simulink model "s_c856m4k"  (R2016b)
settings: Solver=VariableStepAuto  StartTime=0.0  StopTime=10  RelTol=1e-3  EnableMultiTasking=on
undefined symbols (not defined in the file): fft_stages
libraries: xbsIndex_r4 x11811, casper_library_misc x54, casper_library_scopes x5, xps_library x2
(part 25 of 92)

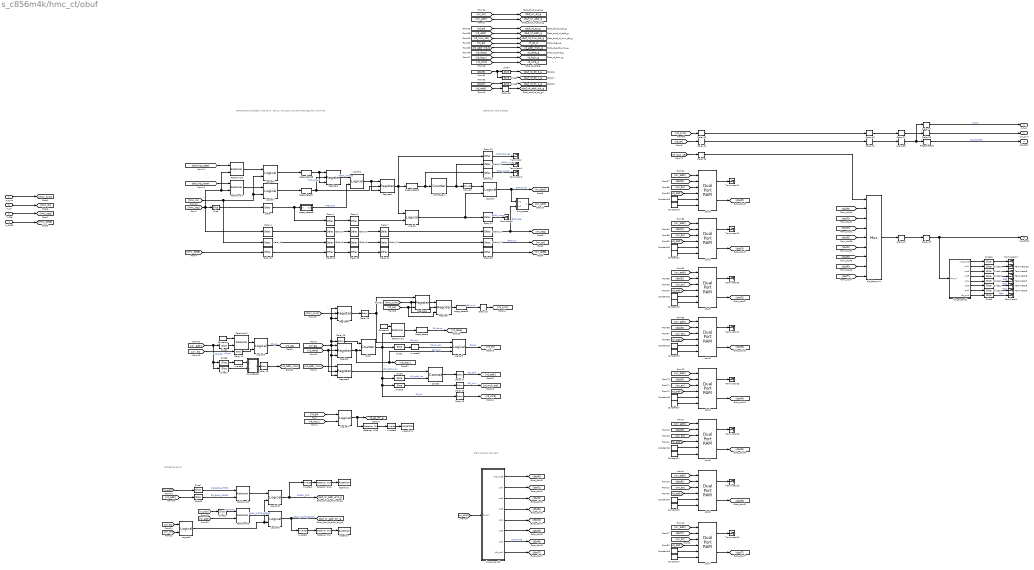
== system s_c856m4k/hmc_ct/obuf ==
  note: Addressing errors
  note: Eight parallel channels.
  note: Create the write address.
  note: Generate the corrected write bank - taking into account
      | out-of-order tags from the HMC.
  in_sync : Inport
  in_dv : Inport  Port=2
  in_tag : Inport  Port=3
  in_d256 : Inport  Port=4
  Assertion : Assertion
  Assertion1 : Assertion
  Assertion2 : Assertion
  Concat : xbsIndex_r4/Concat  num_inputs=2  dbl_ovrd=off  block_type=concat
  Constant1 : xbsIndex_r4/Constant  const=511-32  gui_display_data_type=Fixed-point  arith_type=Unsigned  n_bits=9  bin_pt=0  preci_type=Single  exp_width=8  frac_width=24  explicit_period=on  period=1  equ=P=C  opselect=C  inp2=PCIN>>17  opr=+  inp1=P  carry=CIN  dbl_ovrd=off  block_type=constant
  Constant{10,14,16,18,20,22,24,26} (8 alike) : xbsIndex_r4/Constant  const=0  gui_display_data_type=Fixed-point  arith_type=Unsigned  n_bits=256  bin_pt=0  preci_type=Single  exp_width=8  frac_width=24  explicit_period=on  period=1  equ=P=C  opselect=C  inp2=PCIN>>17  opr=+  inp1=P  carry=CIN  dbl_ovrd=off  block_type=constant
  Constant{11,15,17,19,21,23,25,27} (8 alike) : xbsIndex_r4/Constant  const=0  gui_display_data_type=Boolean  arith_type=Boolean  n_bits=256  bin_pt=0  preci_type=Single  exp_width=8  frac_width=24  explicit_period=on  period=1  equ=P=C  opselect=C  inp2=PCIN>>17  opr=+  inp1=P  carry=CIN  dbl_ovrd=off  block_type=constant
  Constant4 : xbsIndex_r4/Constant  const=0  gui_display_data_type=Fixed-point  arith_type=Unsigned  n_bits=8  bin_pt=0  preci_type=Single  exp_width=8  frac_width=24  explicit_period=on  period=1  equ=P=C  opselect=C  inp2=PCIN>>17  opr=+  inp1=P  carry=CIN  dbl_ovrd=off  block_type=constant
  Convert : xbsIndex_r4/Convert  gui_display_data_type=Boolean  arith_type=Boolean  n_bits=16  bin_pt=14  float_type=Single  exp_bits=8  fraction_bits=24  quantization=Truncate  overflow=Wrap  en=off  latency=0  pipeline=off  dbl_ovrd=off  block_type=convert
  Delay{,3..4,31} (4 alike) : xbsIndex_r4/Delay  rst=off  infoeditControl=Selection of Reset will increase slice count due to use of real FFs and instead of SRLs  en=off  latency=3  reg_retiming=off  dbl_ovrd=off  block_type=delay
      settings: infoedit=Hardware notes: A delay line is a chain, each link of which is an SRL16 or SRL32 followed by a flip-flop.
  Delay{1..2,5..12,14..23,27..29,32..35,37..38,40,45} (31 alike) : xbsIndex_r4/Delay  rst=off  infoeditControl=Selection of Reset will increase slice count due to use of real FFs and instead of SRLs  en=off  latency=1  reg_retiming=off  dbl_ovrd=off  block_type=delay
      settings: infoedit=Hardware notes: A delay line is a chain, each link of which is an SRL16 or SRL32 followed by a flip-flop.
  Delay13 : xbsIndex_r4/Delay  rst=off  infoeditControl=Selection of Reset will increase slice count due to use of real FFs and instead of SRLs  en=off  latency=2  reg_retiming=off  dbl_ovrd=off  block_type=delay
      settings: infoedit=Hardware notes: A delay line is a chain, each link of which is an SRL16 or SRL32 followed by a flip-flop.
  Delay25 : xbsIndex_r4/Delay  rst=off  infoeditControl=Selection of Reset will increase slice count due to use of real FFs and instead of SRLs  en=off  latency=pkt_buffer_latency  reg_retiming=off  dbl_ovrd=off  block_type=delay
      settings: infoedit=Hardware notes: A delay line is a chain, each link of which is an SRL16 or SRL32 followed by a flip-flop.
  Delay26 : xbsIndex_r4/Delay  rst=off  infoeditControl=Selection of Reset will increase slice count due to use of real FFs and instead of SRLs  en=off  latency=omux_latency  reg_retiming=off  dbl_ovrd=off  block_type=delay
      settings: infoedit=Hardware notes: A delay line is a chain, each link of which is an SRL16 or SRL32 followed by a flip-flop.
  Delay36 : xbsIndex_r4/Delay  rst=off  infoeditControl=Selection of Reset will increase slice count due to use of real FFs and instead of SRLs  en=off  latency=pkt_buffer_latency  reg_retiming=off  dbl_ovrd=off  block_type=delay
      settings: infoedit=Hardware notes: A delay line is a chain, each link of which is an SRL16 or SRL32 followed by a flip-flop.
  Delay42 : xbsIndex_r4/Delay  rst=off  infoeditControl=Selection of Reset will increase slice count due to use of real FFs and instead of SRLs  en=off  latency=pkt_buffer_latency  reg_retiming=off  dbl_ovrd=off  block_type=delay
      settings: infoedit=Hardware notes: A delay line is a chain, each link of which is an SRL16 or SRL32 followed by a flip-flop.
  Delay43 : xbsIndex_r4/Delay  rst=off  infoeditControl=Selection of Reset will increase slice count due to use of real FFs and instead of SRLs  en=off  latency=omux_latency  reg_retiming=off  dbl_ovrd=off  block_type=delay
      settings: infoedit=Hardware notes: A delay line is a chain, each link of which is an SRL16 or SRL32 followed by a flip-flop.
  Delay46 : xbsIndex_r4/Delay  rst=off  infoeditControl=Selection of Reset will increase slice count due to use of real FFs and instead of SRLs  en=off  latency=27  reg_retiming=off  dbl_ovrd=off  block_type=delay
      settings: infoedit=Hardware notes: A delay line is a chain, each link of which is an SRL16 or SRL32 followed by a flip-flop.
  Gateway Out : xbsIndex_r4/Gateway Out  inherit_from_input=off  hdl_port=off  rows=1  columns=1  UseAsDAC=off  DACChannel='1'  interface=None  automatic_assignment=on  address_offset=hex2dec('00')  intf_name=''  intf_description=''  timing_constraint=None  locs_specified=off  LOCs={}  io_standard={}  block_type=gatewayout
  Gateway Out1 : xbsIndex_r4/Gateway Out  inherit_from_input=off  hdl_port=off  rows=1  columns=1  UseAsDAC=off  DACChannel='1'  interface=None  automatic_assignment=on  address_offset=hex2dec('00')  intf_name=''  intf_description=''  timing_constraint=None  locs_specified=off  LOCs={}  io_standard={}  block_type=gatewayout
  Gateway Out2 : xbsIndex_r4/Gateway Out  inherit_from_input=off  hdl_port=off  rows=1  columns=1  UseAsDAC=off  DACChannel='1'  interface=None  automatic_assignment=on  address_offset=hex2dec('00')  intf_name=''  intf_description=''  timing_constraint=None  locs_specified=off  LOCs={}  io_standard={}  block_type=gatewayout
  Inverter{2..6} (5 alike) : xbsIndex_r4/Inverter  en=off  latency=0  dbl_ovrd=off  block_type=inv
  Logical{,1,3..4} (4 alike) : xbsIndex_r4/Logical  logical_function=AND  inputs=2  en=off  latency=1  precision=Full  arith_type=Unsigned  n_bits=16  bin_pt=0  align_bp=on  dbl_ovrd=off  block_type=logical
  Logical10 : xbsIndex_r4/Logical  logical_function=AND  inputs=2  en=off  latency=0  precision=Full  arith_type=Unsigned  n_bits=16  bin_pt=0  align_bp=on  dbl_ovrd=off  block_type=logical
  Logical2 : xbsIndex_r4/Logical  logical_function=XOR  inputs=2  en=off  latency=1  precision=Full  arith_type=Unsigned  n_bits=16  bin_pt=0  align_bp=on  dbl_ovrd=off  block_type=logical
  Logical5 : xbsIndex_r4/Logical  logical_function=AND  inputs=3  en=off  latency=1  precision=Full  arith_type=Unsigned  n_bits=16  bin_pt=0  align_bp=on  dbl_ovrd=off  block_type=logical
  Logical6 : xbsIndex_r4/Logical  logical_function=AND  inputs=2  en=off  latency=3  precision=Full  arith_type=Unsigned  n_bits=16  bin_pt=0  align_bp=on  dbl_ovrd=off  block_type=logical
  Logical7 : xbsIndex_r4/Logical  logical_function=AND  inputs=2  en=off  latency=3  precision=Full  arith_type=Unsigned  n_bits=16  bin_pt=0  align_bp=on  dbl_ovrd=off  block_type=logical
  Logical8 : xbsIndex_r4/Logical  logical_function=AND  inputs=2  en=off  latency=0  precision=Full  arith_type=Unsigned  n_bits=16  bin_pt=0  align_bp=on  dbl_ovrd=off  block_type=logical
  Logical9 : xbsIndex_r4/Logical  logical_function=AND  inputs=2  en=off  latency=0  precision=Full  arith_type=Unsigned  n_bits=16  bin_pt=0  align_bp=on  dbl_ovrd=off  block_type=logical
  Register{,1..4,6..7} (7 alike) : xbsIndex_r4/Register  init=0  rst=on  en=on  dbl_ovrd=off  block_type=register
  Relational1 : xbsIndex_r4/Relational  mode=a=b  op_type=Bool  en=off  latency=1  dbl_ovrd=off  block_type=relational
  Relational2 : xbsIndex_r4/Relational  mode=a=b  op_type=Bool  en=off  latency=1  dbl_ovrd=off  block_type=relational
  Relational{3,5..7} (4 alike) : xbsIndex_r4/Relational  mode=a=b  op_type=Bool  en=off  latency=0  dbl_ovrd=off  block_type=relational
  Slice : xbsIndex_r4/Slice  nbits=1  boolean_output=on  mode=Upper Bit Location + Width  bit1=0  base1=MSB of Input  bit0=0  base0=LSB of Input  dbl_ovrd=off  block_type=slice
  Slice1 : xbsIndex_r4/Slice  nbits=1  boolean_output=on  mode=Lower Bit Location + Width  bit1=0  base1=MSB of Input  bit0=5  base0=LSB of Input  dbl_ovrd=off  block_type=slice
  Slice{9..16} (8 alike) : xbsIndex_r4/Slice  nbits=9  boolean_output=off  mode=Lower Bit Location + Width  bit1=0  base1=MSB of Input  bit0=0  base0=LSB of Input  dbl_ovrd=off  block_type=slice
  Slice17 : xbsIndex_r4/Slice  nbits=1  boolean_output=off  mode=Upper Bit Location + Width  bit1=-1  base1=MSB of Input  bit0=0  base0=LSB of Input  dbl_ovrd=off  block_type=slice
  Slice18 : xbsIndex_r4/Slice  nbits=2  boolean_output=off  mode=Upper Bit Location + Width  bit1=0  base1=MSB of Input  bit0=8 - 3  base0=LSB of Input  dbl_ovrd=off  block_type=slice
  Slice19 : xbsIndex_r4/Slice  nbits=3  boolean_output=off  mode=Lower Bit Location + Width  bit1=0  base1=MSB of Input  bit0=5+1  base0=LSB of Input  dbl_ovrd=off  block_type=slice
  Slice2 : xbsIndex_r4/Slice  nbits=8  boolean_output=off  mode=Lower Bit Location + Width  bit1=0  base1=MSB of Input  bit0=0  base0=LSB of Input  dbl_ovrd=off  block_type=slice
  Slice21 : xbsIndex_r4/Slice  nbits=1  boolean_output=off  mode=Two Bit Locations  bit1=0  base1=MSB of Input  bit0=3  base0=LSB of Input  dbl_ovrd=off  block_type=slice
  Slice3 : xbsIndex_r4/Slice  nbits=5  boolean_output=off  mode=Lower Bit Location + Width  bit1=0  base1=MSB of Input  bit0=0  base0=LSB of Input  dbl_ovrd=off  block_type=slice
  Slice4 : xbsIndex_r4/Slice  nbits=12  boolean_output=off  mode=Lower Bit Location + Width  bit1=0  base1=MSB of Input  bit0=0  base0=LSB of Input  dbl_ovrd=off  block_type=slice
  Slice5 : xbsIndex_r4/Slice  nbits=12  boolean_output=off  mode=Lower Bit Location + Width  bit1=0  base1=MSB of Input  bit0=32*7  base0=LSB of Input  dbl_ovrd=off  block_type=slice
  Slice6 : xbsIndex_r4/Slice  nbits=12  boolean_output=off  mode=Lower Bit Location + Width  bit1=0  base1=MSB of Input  bit0=32  base0=LSB of Input  dbl_ovrd=off  block_type=slice
  Slice7 : xbsIndex_r4/Slice  nbits=2  boolean_output=off  mode=Upper Bit Location + Width  bit1=0  base1=MSB of Input  bit0=0  base0=LSB of Input  dbl_ovrd=off  block_type=slice
  Slice8 : xbsIndex_r4/Slice  nbits=1  boolean_output=off  mode=Upper Bit Location + Width  bit1=0  base1=MSB of Input  bit0=0  base0=LSB of Input  dbl_ovrd=off  block_type=slice
  Terminator{,1..19} (20 alike) : Terminator
  WRITE_bank : xbsIndex_r4/Counter  cnt_type=Free Running  cnt_to=Inf  operation=Up  start_count=0  cnt_by_val=1  arith_type=Unsigned  n_bits=1  bin_pt=0  load_pin=off  rst=off  en=on  explicit_period=on  period=1  use_behavioral_HDL=off  implementation=Fabric  dbl_ovrd=off  block_type=counter
  bus_create : Subsystem  AncestorBlock=casper_library_flow_control/bus_create  mask(bus_create){inputNum=2}
      mask prompts: inputNum "Number of inputs:"
      mask init:
      | bus_create_init(gcb,...
      |     'inputNum', inputNum);
  bus_create1 : Subsystem  AncestorBlock=casper_library_flow_control/bus_create  mask(bus_create){inputNum=2}
      mask prompts: inputNum "Number of inputs:"
      mask init:
      | bus_create_init(gcb,...
      |     'inputNum', inputNum);
  bus_expand2 : Subsystem  AncestorBlock=casper_library_flow_control/bus_expand  mask(bus_expand){mode=divisions of equal size, outputNum=8, outputWidth=32, outputBinaryPt=0, outputArithmeticType=0, show_format=on, outputToWorkspace=off, variablePrefix=out, outputToModelAsWell=on}
      mask prompts: outputNum "Number of outputs:"; outputWidth "Output width:"; outputBinaryPt "Output binary point position:"; outputArithmeticType "Output arithmetic type (ufix=0, fix=1, bool=2):"; show_format "Print format string?"; outputToWorkspace "Output to workspace?"; variablePrefix "Variable name prefix:"; outputToModelAsWell "Output to model as well?"
      mask help:
      | Expands a 'bus' made using a bus_create or Xilinx
      | concat block.
      | The input will be divided into the specified number
      | of outputs with the specified arithmetic types.
      | Divisions are made from most significant bit.
      mask init: same as s_c856m4k/bus_expand
      settings: AttributesFormatString=8 outputs: uf32.0,uf32.0,uf32.0,uf32.0,uf32.0,uf32.0,uf32.0,uf32.0,
      mask TypeOptions mode: divisions of equal size | divisions of arbitrary size
      mask Callback mode: bus_expand_callback();
      mask Callback outputWidth: bus_expand_callback();
      mask Callback outputToWorkspace: bus_expand_callback();
  bus_expand3 : Subsystem  AncestorBlock=casper_library_flow_control/bus_expand  mask(bus_expand){mode=divisions of equal size, outputNum=8, outputWidth=32, outputBinaryPt=0, outputArithmeticType=0, show_format=off, outputToWorkspace=off, variablePrefix=out, outputToModelAsWell=on}
      mask prompts: outputNum "Number of outputs:"; outputWidth "Output width:"; outputBinaryPt "Output binary point position:"; outputArithmeticType "Output arithmetic type (ufix=0, fix=1, bool=2):"; show_format "Print format string?"; outputToWorkspace "Output to workspace?"; variablePrefix "Variable name prefix:"; outputToModelAsWell "Output to model as well?"
      mask help:
      | Expands a 'bus' made using a bus_create or Xilinx
      | concat block.
      | The input will be divided into the specified number
      | of outputs with the specified arithmetic types.
      | Divisions are made from most significant bit.
      mask init: same as s_c856m4k/bus_expand
      settings: AttributesFormatString=8 outputs
      mask TypeOptions mode: divisions of equal size | divisions of arbitrary size
      mask Callback mode: bus_expand_callback();
      mask Callback outputWidth: bus_expand_callback();
      mask Callback outputToWorkspace: bus_expand_callback();
  edge_detect{,1,3,6..8} (6 alike) : casper_library_misc/edge_detect  edge=Rising  polarity=Active High  x_in=[0 0.08 0.08 0.16 0.16 0.24 0.24 0.32 0.32 0.4]  y_in="[-1 -1  1  1  1  1  1  1  1  1]"  x_out=[0.6 0.68 0.68 0.76 0.76 0.84 0.84 0.92 0.92 1]  y_out="[-1 -1  1  1 -1 -1 -1 -1 -1 -1]"
  edge_detect5 : Subsystem  AncestorBlock=casper_library_misc/edge_detect  mask(edge_detect){edge=Falling, polarity=Active High, x_in=[0 0.08 0.08 0.16 0.16 0.24 0.24 0.32 0.32 0.4], y_in=[-1 -1  1  1  1  1  1  1  1  1], x_out=[0.6 0.68 0.68 0.76 0.76 0.84 0.84 0.92 0.92 1], y_out=[-1 -1  1  1 -1 -1 -1 -1 -1 -1]}
      mask prompts: edge "Edge Type"; polarity "Output Polarity"; x_in "Input X Positions"; y_in "Input Y Positions"; x_out "Output X Positions"; y_out "Output Y Positions"
      mask help: Output is active for one-cycle after each edge of the specified type (i.e. rising, falling or both).
      mask init: same as s_c856m4k/edge_detect1
      settings: AttributesFormatString=|
      | falling edges
      | active high
      mask Help: Output is active for one-cycle after each edge of the specified type (i.e. rising, falling, or both).  Latency is zero.
      mask TypeOptions edge: Rising | Falling | Both
      mask TypeOptions polarity: Active High | Active Low
      mask Display:
      | plot(x_in_num,0.5+y_in_num*0.2);
      | plot(x_out_num,0.5+y_out_num*0.2);
  obuf{0..7} (8 alike) : xbsIndex_r4/Dual Port RAM  depth=2^(output_len_bits + 2)  initVector=zeros(1, 2^(output_len_bits + 2))  distributed_mem=Block RAM  init_a=0  init_b=0  rst_a=off  rst_b=off  en_a=off  en_b=off  latency=pkt_buffer_latency  write_mode_A=Read After Write  write_mode_B=Read After Write  optimize=Area  dbl_ovrd=off  block_type=dpram
  pkt_data_mux : xbsIndex_r4/Mux  inputs=8  en=off  latency=omux_latency  precision=Full  arith_type=Unsigned  n_bits=16  bin_pt=14  quantization=Truncate  overflow=Wrap  dbl_ovrd=off  block_type=mux
  rd_ctr : xbsIndex_r4/Counter  cnt_type=Free Running  cnt_to=Inf  operation=Up  start_count=0  cnt_by_val=1  arith_type=Unsigned  n_bits=9  bin_pt=0  load_pin=off  rst=on  en=on  explicit_period=on  period=1  use_behavioral_HDL=off  implementation=Fabric  dbl_ovrd=off  block_type=counter
  out_sync : Outport
  out_dv : Outport  Port=2
  out_d256 : Outport  Port=3
  pkt_start : Outport  Port=4
  tag scope: obuf_ct_addr_err2_g=global, obuf_ct_addr_err_g=global, obuf_rd_addr_g=global, obuf_rd_addr_out_g=global, obuf_rd_d0_0_g=global, obuf_rd_d0_7_g=global, obuf_rd_d7_1_g=global, obuf_rd_en_g=global, obuf_rd_mux_sel_g=global, obuf_wr_addr_g=global, obuf_wr_en_g=global, rd_addr_msw_g=global, rd_busy_g=global, rd_ctr9_g=global, rd_done_g=global, rd_go_err_g=global, rd_go_g=global
  wires:
  Delay28/1 -> out_sync/1
  Delay27/1 -> Delay28/1
  Delay26/1 -> Delay27/1
  Delay25/1 -> Delay26/1
  [rd_sync] -> Delay25/1
  Delay29/1 -> [rd_sync]
  [rd_go] -> Register6/3, Register7/3
  [hmc_sync] -> Register6/2, Register7/2
  edge_detect3/1 -> Delay29/1  "RD_sync"
  Register7/1 -> edge_detect3/1
  Register6/1 -> Register7/1
  Delay19/1 -> Logical5/1, Register6/1  "RD_arm"
  Register4/1 -> Delay19/1
  [hmc_sync] -> Register4/2
  Gateway Out2/1 -> Inverter6/1
  Inverter6/1 -> Assertion2/1
  [rd_en] -> [obuf_rd_en_g]
  Delay15/1 -> [rd_ctr9]
  [rd_ctr9] -> [rd_ctr9_g]
  [rd_busy] -> [rd_busy_g]
  [rd_done] -> [rd_done_g]
  [rd_addr_msw] -> [rd_addr_msw_g]
  [rd_go] -> [rd_go_g]
  Slice19/1 -> Delay18/1
  Delay18/1 -> [rd_mux_sel]  "RD_mux"
  Delay17/1 -> [rd_addr]  "RD_addr"
  Logical5/1 -> [rd_en]  "RD_en"
  Concat/1 -> Delay17/1
  [rd_done] -> Register/2, Register3/2
  edge_detect/1 -> [rd_done]  "RD_done"
  Relational1/1 -> edge_detect/1
  Constant1/1 -> Relational1/1
  Register3/1 -> Concat/1  "RD_addr_msw"
  [rd_addr_msw] -> Register3/1
  Slice3/1 -> Concat/2  "RD_addr_lsw"
  Inverter5/1 -> Logical5/2  "RD_en_raw"
  Slice1/1 -> Inverter5/1
  rd_ctr/1 -> Relational1/2, Slice3/1, Slice19/1, Delay15/1, Slice1/1  "RD_ctr"
  Delay16/1 -> rd_ctr/1
  Register/1 -> [rd_busy], Logical5/3, rd_ctr/2  "RD_busy"
  [rd_go] -> Register/1, Register/3, Register3/3, Delay16/1, Register4/1, Register4/3
  Logical4/1 -> [rd_go_err_g], Gateway Out2/1
  [rd_busy] -> Logical4/2
  [rd_go] -> Logical4/1
  Delay13/1 -> [rd_addr_msw]
  Logical3/1 -> [rd_go]  "RD_go"
  Delay14/1 -> Logical3/2
  Slice17/1 -> bus_create1/2(in2)
  Inverter3/1 -> bus_create1/1(in1)
  bus_create1/1(bus_out) -> Delay13/1
  Slice8/1 -> Inverter3/1
  [wr_addr] -> Slice17/1, Slice8/1, Slice2/1  "WR_addr"
  Slice2/1 -> Relational2/2
  [wr_en] -> Delay14/1  "WR_en"
  Relational2/1 -> Logical3/1
  Constant4/1 -> Relational2/1
  Delay46/1 -> [obuf_rd_addr_out_g]
  [rd_addr] -> Delay46/1
  Slice6/1 -> [obuf_rd_d7_1_g]
  [obuf7] -> Slice6/1
  Slice5/1 -> [obuf_rd_d0_7_g]
  Slice4/1 -> [obuf_rd_d0_0_g]
  [obuf0] -> Slice4/1, Slice5/1
  [rd_mux_sel] -> [obuf_rd_mux_sel_g]
  [rd_addr] -> [obuf_rd_addr_g]
  [wr_addr] -> [obuf_wr_addr_g]
  [wr_en] -> [obuf_wr_en_g]
  Inverter4/1 -> Gateway Out1/1
  Gateway Out1/1 -> Assertion1/1
  Logical10/1 -> [obuf_ct_addr_err2_g], Inverter4/1  "CHECK_DIFF"
  Relational5/1 -> Logical8/1  "READ_WRITE_ERROR"
  Relational3/1 -> Logical10/1
  Slice18/1 -> Relational3/2  "RD_BANK_CHECK"
  Slice7/1 -> Relational3/1  "WR_BANK_CHECK"
  [rd_addr] -> Slice18/1
  [wr_addr] -> Slice7/1
  Logical9/1 -> Logical8/2, Logical10/2
  Slice21/1 -> Relational5/1  "WADDR7"
  Inverter2/1 -> Gateway Out/1
  Gateway Out/1 -> Assertion/1
  [wr_en] -> Logical9/2
  [rd_en] -> Logical9/1
  Logical8/1 -> Inverter2/1, [obuf_ct_addr_err_g]  "READ_WRITE_ERROR"
  [rd_addr] -> Relational5/2
  [wr_addr] -> Slice21/1
  bus_expand3/8(lsb_out1) -> [dbuf7]
  bus_expand3/7(out2) -> [dbuf6]  "DATA_TAG"
  bus_expand3/6(out3) -> [dbuf5]
  bus_expand3/5(out4) -> [dbuf4]
  bus_expand3/4(out5) -> [dbuf3]
  bus_expand3/3(out6) -> [dbuf2]
  bus_expand3/2(out7) -> [dbuf1]
  bus_expand3/1(msb_out8) -> [dbuf0]
  [wr_d256] -> bus_expand3/1(bus_in)
  Delay40/1 -> Delay45/1
  Delay38/1 -> edge_detect1/1, Delay37/1
  Delay37/1 -> out_dv/1  "out_dv"
  Delay45/1 -> bus_expand2/1(bus_in), out_d256/1
  edge_detect1/1 -> pkt_start/1  "out_pkt_start"
  Delay43/1 -> Delay38/1
  Delay42/1 -> Delay43/1
  [rd_en] -> Delay42/1
  Delay36/1 -> pkt_data_mux/1
  [obuf1] -> pkt_data_mux/3
  [obuf0] -> pkt_data_mux/2
  [obuf2] -> pkt_data_mux/4
  [obuf3] -> pkt_data_mux/5
  [obuf7] -> pkt_data_mux/9
  [obuf5] -> pkt_data_mux/7
  [obuf6] -> pkt_data_mux/8
  [obuf4] -> pkt_data_mux/6
  [rd_mux_sel] -> Delay36/1
  obuf4/1 -> Terminator15/1
  obuf4/2 -> [obuf4]
  Constant27/1 -> obuf4/6
  Constant26/1 -> obuf4/5
  [rd_addr] -> obuf4/4
  [wr_en] -> obuf4/3
  [wr_addr] -> obuf4/1
  [dbuf4] -> obuf4/2
  obuf3/1 -> Terminator14/1
  obuf3/2 -> [obuf3]
  Constant25/1 -> obuf3/6
  Constant24/1 -> obuf3/5
  [rd_addr] -> obuf3/4
  [wr_en] -> obuf3/3
  [wr_addr] -> obuf3/1
  [dbuf3] -> obuf3/2
  obuf2/1 -> Terminator13/1
  obuf2/2 -> [obuf2]
  Constant23/1 -> obuf2/6
  Constant22/1 -> obuf2/5
  [rd_addr] -> obuf2/4
  [wr_en] -> obuf2/3
  [wr_addr] -> obuf2/1
  [dbuf2] -> obuf2/2
  obuf1/1 -> Terminator12/1
  obuf1/2 -> [obuf1]
  Constant21/1 -> obuf1/6
  Constant20/1 -> obuf1/5
  [rd_addr] -> obuf1/4
  [wr_en] -> obuf1/3
  [wr_addr] -> obuf1/1
  [dbuf1] -> obuf1/2
  obuf0/1 -> Terminator11/1
  obuf0/2 -> [obuf0]
  Constant19/1 -> obuf0/6
  Constant18/1 -> obuf0/5
  [rd_addr] -> obuf0/4
  [wr_en] -> obuf0/3
  [wr_addr] -> obuf0/1
  [dbuf0] -> obuf0/2
  obuf7/1 -> Terminator10/1
  obuf7/2 -> [obuf7]
  Constant17/1 -> obuf7/6
  Constant16/1 -> obuf7/5
  [rd_addr] -> obuf7/4
  [wr_en] -> obuf7/3
  [wr_addr] -> obuf7/1
  [dbuf7] -> obuf7/2
  obuf6/1 -> Terminator19/1
  obuf6/2 -> [obuf6]
  Constant15/1 -> obuf6/6
  Constant14/1 -> obuf6/5
  [rd_addr] -> obuf6/4
  [wr_en] -> obuf6/3
  [wr_addr] -> obuf6/1
  [dbuf6] -> obuf6/2
  pkt_data_mux/1 -> Delay40/1
  obuf5/1 -> Terminator18/1
  obuf5/2 -> [obuf5]
  bus_expand2/4(out5) -> Slice13/1
  Slice13/1 -> Terminator8/1
  Slice14/1 -> Terminator9/1
  Slice15/1 -> Terminator16/1
  Slice16/1 -> Terminator17/1
  bus_expand2/3(out6) -> Slice14/1
  bus_expand2/2(out7) -> Slice15/1
  bus_expand2/1(msb_out8) -> Slice16/1
  Slice9/1 -> Terminator4/1  "tag0"
  Slice10/1 -> Terminator5/1  "tag1"
  Slice11/1 -> Terminator6/1  "tag2"
  Slice12/1 -> Terminator7/1  "tag3"
  bus_expand2/5(out4) -> Slice12/1
  bus_expand2/6(out3) -> Slice11/1
  bus_expand2/7(out2) -> Slice10/1
  bus_expand2/8(lsb_out1) -> Slice9/1
  Constant11/1 -> obuf5/6
  Constant10/1 -> obuf5/5
  [rd_addr] -> obuf5/4
  [wr_en] -> obuf5/3
  [wr_addr] -> obuf5/1
  [dbuf5] -> obuf5/2
  Delay35/1 -> [wr_d256]
  Delay34/1 -> Delay35/1
  Delay33/1 -> Delay34/1
  Delay32/1 -> Delay33/1
  Delay31/1 -> Delay32/1
  [hmc_d256] -> Delay31/1
  in_d256/1 -> [hmc_d256]
  edge_detect8/1 -> WRITE_bank/1, Delay21/1
  Register1/1 -> edge_detect8/1, Logical/1, Delay23/1
  Delay23/1 -> Terminator/1  "BANK_change"
  Delay22/1 -> Terminator3/1  "BANK_wrong"
  Delay21/1 -> Terminator2/1  "BANK_switch"
  Delay20/1 -> Terminator1/1  "BANK_wr_raw"
  Delay3/1 -> Delay8/1
  Delay8/1 -> Delay9/1
  Delay9/1 -> Delay10/1
  Delay10/1 -> Delay11/1
  Delay11/1 -> [wr_en]  "BANK_dv"
  Delay12/1 -> bus_create/2(in2), [wr_tag]  "BANK_tag"
  bus_create/1(bus_out) -> [wr_addr]
  Logical2/1 -> bus_create/1(in1), [wr_bank]  "BANK_final"
  Delay2/1 -> Logical/2
  Logical/1 -> Logical2/2, Delay22/1
  Delay7/1 -> Delay12/1
  Delay6/1 -> Delay7/1
  Delay5/1 -> Delay6/1
  Delay4/1 -> Delay5/1
  Convert/1 -> Logical2/1
  Delay1/1 -> Delay2/1
  WRITE_bank/1 -> Convert/1, Delay20/1
  Logical1/1 -> Register1/1, Register1/3
  Register2/1 -> Logical1/1  "BANK_change"
  edge_detect7/1 -> Register2/2, Register1/2
  [hmc_dv] -> Delay3/1, Logical7/2, Logical6/2
  [obuf_trig_lower] -> Relational7/1
  edge_detect6/1 -> Register2/1, Register2/3  "TAG_upper"
  Relational6/1 -> Logical6/1
  [obuf_trig_upper] -> Relational6/1
  Delay/1 -> edge_detect5/1(in), Delay1/1
  edge_detect5/1(out) -> Logical1/2  "TAG_drop"
  Slice/1 -> Delay/1
  [hmc_tag] -> Slice/1, Delay4/1, Relational7/2, Relational6/2
  in_sync/1 -> [hmc_sync]
  in_tag/1 -> [hmc_tag]
  in_dv/1 -> [hmc_dv]
  Relational7/1 -> Logical7/1
  Logical6/1 -> edge_detect6/1
  Logical7/1 -> edge_detect7/1

== system s_c856m4k/hmc_ct/read_map_gen_interleave ==
  note: collection of like channels
  note: Straight collection, no x-interleave
  note: x-interleave, SLICED
  note: x-interleave, CALCED
  note: compare calculated to sliced
  addr : Inport
  num_x : Inport  Port=2
  one_over_num_x : Inport  Port=3
  chans_per_x_div8 : Inport  Port=4
  AddSub2 : xbsIndex_r4/AddSub  mode=Subtraction  use_carryin=off  use_carryout=off  en=off  latency=0  precision=Full  arith_type=Unsigned  n_bits=7  bin_pt=0  quantization=Truncate  overflow=Wrap  use_behavioral_HDL=off  hw_selection=Fabric  pipelined=off  dbl_ovrd=off  block_type=addsub
  AddSub3 : xbsIndex_r4/AddSub  mode=Subtraction  use_carryin=off  use_carryout=off  en=off  latency=3  precision=User Defined  arith_type=Unsigned  n_bits=in_vec_bits - 2  bin_pt=0  quantization=Truncate  overflow=Wrap  use_behavioral_HDL=off  hw_selection=Fabric  pipelined=off  dbl_ovrd=off  block_type=addsub
  AddSub4 : xbsIndex_r4/AddSub  mode=Addition  use_carryin=off  use_carryout=off  en=off  latency=3  precision=User Defined  arith_type=Unsigned  n_bits=in_vec_bits  bin_pt=0  quantization=Truncate  overflow=Wrap  use_behavioral_HDL=off  hw_selection=Fabric  pipelined=off  dbl_ovrd=off  block_type=addsub
  Assert1 : xbsIndex_r4/Assert  assert_type=on  type_source=Explicitly  gui_display_data_type=Fixed-point  arith_type=Unsigned  n_bits=in_vec_bits  bin_pt=0  preci_type=Single  exp_width=8  frac_width=24  assert_rate=on  rate_source=Explicitly  period=1  output_port=on  block_type=assert
  Assert{2,6..9} (5 alike) : xbsIndex_r4/Assert  assert_type=on  type_source=Explicitly  gui_display_data_type=Fixed-point  arith_type=Unsigned  n_bits=in_vec_bits + out_vec_bits + 1  bin_pt=0  preci_type=Single  exp_width=8  frac_width=24  assert_rate=on  rate_source=Explicitly  period=1  output_port=on  block_type=assert
  Assert3 : xbsIndex_r4/Assert  assert_type=on  type_source=Explicitly  gui_display_data_type=Fixed-point  arith_type=Unsigned  n_bits=8  bin_pt=0  preci_type=Single  exp_width=8  frac_width=24  assert_rate=on  rate_source=Explicitly  period=1  output_port=on  block_type=assert
  Assert4 : xbsIndex_r4/Assert  assert_type=on  type_source=Explicitly  gui_display_data_type=Fixed-point  arith_type=Unsigned  n_bits=9  bin_pt=8  preci_type=Single  exp_width=8  frac_width=24  assert_rate=on  rate_source=Explicitly  period=1  output_port=on  block_type=assert
  Assert5 : xbsIndex_r4/Assert  assert_type=on  type_source=Explicitly  gui_display_data_type=Fixed-point  arith_type=Unsigned  n_bits=12  bin_pt=0  preci_type=Single  exp_width=8  frac_width=24  assert_rate=on  rate_source=Explicitly  period=1  output_port=on  block_type=assert
  Assertion : Assertion
  Concat1 : xbsIndex_r4/Concat  num_inputs=3  dbl_ovrd=off  block_type=concat
  Concat10 : xbsIndex_r4/Concat  num_inputs=3  dbl_ovrd=off  block_type=concat
  Concat4 : xbsIndex_r4/Concat  num_inputs=3  dbl_ovrd=off  block_type=concat
  Concat8 : xbsIndex_r4/Concat  num_inputs=2  dbl_ovrd=off  block_type=concat
  Mult3 : xbsIndex_r4/Mult  precision=User Defined  arith_type=Unsigned  n_bits=in_vec_bits - 1 + 8  bin_pt=0  quantization=Truncate  overflow=Wrap  en=off  latency=3  use_behavioral_HDL=off  opt=Speed  use_embedded=on  optimum_pipeline=off  pipeline=on  dbl_ovrd=off  use_rpm=on  placement_style=Triangular  block_type=mult
  Mult4 : xbsIndex_r4/Mult  precision=User Defined  arith_type=Unsigned  n_bits=in_vec_bits + 8  bin_pt=0  quantization=Truncate  overflow=Wrap  en=off  latency=3  use_behavioral_HDL=off  opt=Speed  use_embedded=on  optimum_pipeline=off  pipeline=on  dbl_ovrd=off  use_rpm=on  placement_style=Triangular  block_type=mult
  Mult5 : xbsIndex_r4/Mult  precision=User Defined  arith_type=Unsigned  n_bits=in_vec_bits - 1 + 8  bin_pt=0  quantization=Truncate  overflow=Wrap  en=off  latency=3  use_behavioral_HDL=off  opt=Speed  use_embedded=on  optimum_pipeline=off  pipeline=on  dbl_ovrd=off  use_rpm=on  placement_style=Triangular  block_type=mult
  Relational : xbsIndex_r4/Relational  mode=a=b  op_type=Bool  en=off  latency=0  dbl_ovrd=off  block_type=relational
  Terminator{,1..7} (8 alike) : Terminator
  bank1 : xbsIndex_r4/Slice  nbits=x_bits  boolean_output=off  mode=Upper Bit Location + Width  bit1=0  base1=MSB of Input  bit0=0  base0=LSB of Input  dbl_ovrd=off  block_type=slice
  bank10 : xbsIndex_r4/Slice  nbits=in_vec_bits  boolean_output=off  mode=Lower Bit Location + Width  bit1=2  base1=MSB of Input  bit0=out_vec_bits  base0=LSB of Input  dbl_ovrd=off  block_type=slice
  bank11 : xbsIndex_r4/Slice  nbits=out_vec_bits  boolean_output=off  mode=Lower Bit Location + Width  bit1=2  base1=MSB of Input  bit0=0  base0=LSB of Input  dbl_ovrd=off  block_type=slice
  bank12 : xbsIndex_r4/Slice  nbits=1  boolean_output=off  mode=Upper Bit Location + Width  bit1=0  base1=MSB of Input  bit0=output_len_bits - 1  base0=LSB of Input  dbl_ovrd=off  block_type=slice
  bank2 : xbsIndex_r4/Slice  nbits=x_bits  boolean_output=off  mode=Upper Bit Location + Width  bit1=0  base1=MSB of Input  bit0=0  base0=LSB of Input  dbl_ovrd=off  block_type=slice
  bank23 : xbsIndex_r4/Slice  nbits=x_bits  boolean_output=off  mode=Lower Bit Location + Width  bit1=2  base1=MSB of Input  bit0=0  base0=LSB of Input  dbl_ovrd=off  block_type=slice
  bank25 : xbsIndex_r4/Slice  nbits=x_bits  boolean_output=off  mode=Two Bit Locations  bit1=0  base1=MSB of Input  bit0=x_bits  base0=LSB of Input  dbl_ovrd=off  block_type=slice
  bank3 : xbsIndex_r4/Slice  nbits=out_vec_bits  boolean_output=off  mode=Lower Bit Location + Width  bit1=2  base1=MSB of Input  bit0=in_vec_bits  base0=LSB of Input  dbl_ovrd=off  block_type=slice
  bank4 : xbsIndex_r4/Slice  nbits=out_vec_bits  boolean_output=off  mode=Lower Bit Location + Width  bit1=2  base1=MSB of Input  bit0=in_vec_bits  base0=LSB of Input  dbl_ovrd=off  block_type=slice
  bank5 : xbsIndex_r4/Slice  nbits=in_vec_bits  boolean_output=off  mode=Lower Bit Location + Width  bit1=2  base1=MSB of Input  bit0=0  base0=LSB of Input  dbl_ovrd=off  block_type=slice
  bank6 : xbsIndex_r4/Slice  nbits=in_vec_bits  boolean_output=off  mode=Lower Bit Location + Width  bit1=2  base1=MSB of Input  bit0=0  base0=LSB of Input  dbl_ovrd=off  block_type=slice
  bank7 : xbsIndex_r4/Slice  nbits=x_bits  boolean_output=off  mode=Upper Bit Location + Width  bit1=0  base1=MSB of Input  bit0=0  base0=LSB of Input  dbl_ovrd=off  block_type=slice
  bank8 : xbsIndex_r4/Slice  nbits=out_vec_bits  boolean_output=off  mode=Lower Bit Location + Width  bit1=2  base1=MSB of Input  bit0=in_vec_bits  base0=LSB of Input  dbl_ovrd=off  block_type=slice
  bank9 : xbsIndex_r4/Slice  nbits=in_vec_bits  boolean_output=off  mode=Lower Bit Location + Width  bit1=2  base1=MSB of Input  bit0=0  base0=LSB of Input  dbl_ovrd=off  block_type=slice
  chans_per_x1 : xbsIndex_r4/Constant  const=0  gui_display_data_type=Fixed-point  arith_type=Signed (2's comp)  n_bits=15  bin_pt=0  preci_type=Single  exp_width=8  frac_width=24  explicit_period=on  period=1  equ=P=C  opselect=C  inp2=PCIN>>17  opr=+  inp1=P  carry=CIN  dbl_ovrd=off  block_type=constant
  in_vec_len : xbsIndex_r4/Constant  const=2^in_vec_bits  gui_display_data_type=Fixed-point  arith_type=Unsigned  n_bits=in_vec_bits + 1  bin_pt=0  preci_type=Single  exp_width=8  frac_width=24  explicit_period=on  period=1  equ=P=C  opselect=C  inp2=PCIN>>17  opr=+  inp1=P  carry=CIN  dbl_ovrd=off  block_type=constant
  out_vec_len : xbsIndex_r4/Constant  const=2^out_vec_bits  gui_display_data_type=Fixed-point  arith_type=Unsigned  n_bits=out_vec_bits + 1  bin_pt=0  preci_type=Single  exp_width=8  frac_width=24  explicit_period=on  period=1  equ=P=C  opselect=C  inp2=PCIN>>17  opr=+  inp1=P  carry=CIN  dbl_ovrd=off  block_type=constant
  we_delay1 : Subsystem  AncestorBlock=casper_library_delays/pipeline  mask(pipeline){latency=3}
      mask help:
      | An explicitly laid-out delay line to avoid mapping to SRL16s
      | for use in pipelining to help achieve timing closure.
      mask init:
      | pipeline_init(gcb,'latency',latency);
      settings: AttributesFormatString=Latency = %<latency>
      mask Display:
      | port_label('input', 1, 'd');
      | port_label('output', 1, 'q');
      | disp(['Z^-', num2str(latency)]);
  we_delay10 : Subsystem  AncestorBlock=casper_library_delays/pipeline  mask(pipeline){latency=3}
      mask help:
      | An explicitly laid-out delay line to avoid mapping to SRL16s
      | for use in pipelining to help achieve timing closure.
      mask init:
      | pipeline_init(gcb,'latency',latency);
      settings: AttributesFormatString=Latency = %<latency>
      mask Display:
      | port_label('input', 1, 'd');
      | port_label('output', 1, 'q');
      | disp(['Z^-', num2str(latency)]);
  we_delay11 : Subsystem  AncestorBlock=casper_library_delays/pipeline  mask(pipeline){latency=3}
      mask help:
      | An explicitly laid-out delay line to avoid mapping to SRL16s
      | for use in pipelining to help achieve timing closure.
      mask init:
      | pipeline_init(gcb,'latency',latency);
      settings: AttributesFormatString=Latency = %<latency>
      mask Display:
      | port_label('input', 1, 'd');
      | port_label('output', 1, 'q');
      | disp(['Z^-', num2str(latency)]);
  we_delay12 : Subsystem  AncestorBlock=casper_library_delays/pipeline  mask(pipeline){latency=3}
      mask help:
      | An explicitly laid-out delay line to avoid mapping to SRL16s
      | for use in pipelining to help achieve timing closure.
      mask init:
      | pipeline_init(gcb,'latency',latency);
      settings: AttributesFormatString=Latency = %<latency>
      mask Display:
      | port_label('input', 1, 'd');
      | port_label('output', 1, 'q');
      | disp(['Z^-', num2str(latency)]);
  we_delay13 : Subsystem  AncestorBlock=casper_library_delays/pipeline  mask(pipeline){latency=3}
      mask help:
      | An explicitly laid-out delay line to avoid mapping to SRL16s
      | for use in pipelining to help achieve timing closure.
      mask init:
      | pipeline_init(gcb,'latency',latency);
      settings: AttributesFormatString=Latency = %<latency>
      mask Display:
      | port_label('input', 1, 'd');
      | port_label('output', 1, 'q');
      | disp(['Z^-', num2str(latency)]);
  we_delay14 : Subsystem  AncestorBlock=casper_library_delays/pipeline  mask(pipeline){latency=3}
      mask help:
      | An explicitly laid-out delay line to avoid mapping to SRL16s
      | for use in pipelining to help achieve timing closure.
      mask init:
      | pipeline_init(gcb,'latency',latency);
      settings: AttributesFormatString=Latency = %<latency>
      mask Display:
      | port_label('input', 1, 'd');
      | port_label('output', 1, 'q');
      | disp(['Z^-', num2str(latency)]);
  we_delay15 : Subsystem  AncestorBlock=casper_library_delays/pipeline  mask(pipeline){latency=3}
      mask help:
      | An explicitly laid-out delay line to avoid mapping to SRL16s
      | for use in pipelining to help achieve timing closure.
      mask init:
      | pipeline_init(gcb,'latency',latency);
      settings: AttributesFormatString=Latency = %<latency>
      mask Display:
      | port_label('input', 1, 'd');
      | port_label('output', 1, 'q');
      | disp(['Z^-', num2str(latency)]);
  we_delay16 : Subsystem  AncestorBlock=casper_library_delays/pipeline  mask(pipeline){latency=3}
      mask help:
      | An explicitly laid-out delay line to avoid mapping to SRL16s
      | for use in pipelining to help achieve timing closure.
      mask init:
      | pipeline_init(gcb,'latency',latency);
      settings: AttributesFormatString=Latency = %<latency>
      mask Display:
      | port_label('input', 1, 'd');
      | port_label('output', 1, 'q');
      | disp(['Z^-', num2str(latency)]);
  we_delay17 : Subsystem  AncestorBlock=casper_library_delays/pipeline  mask(pipeline){latency=3}
      mask help:
      | An explicitly laid-out delay line to avoid mapping to SRL16s
      | for use in pipelining to help achieve timing closure.
      mask init:
      | pipeline_init(gcb,'latency',latency);
      settings: AttributesFormatString=Latency = %<latency>
      mask Display:
      | port_label('input', 1, 'd');
      | port_label('output', 1, 'q');
      | disp(['Z^-', num2str(latency)]);
  we_delay18 : Subsystem  AncestorBlock=casper_library_delays/pipeline  mask(pipeline){latency=3}
      mask help:
      | An explicitly laid-out delay line to avoid mapping to SRL16s
      | for use in pipelining to help achieve timing closure.
      mask init:
      | pipeline_init(gcb,'latency',latency);
      settings: AttributesFormatString=Latency = %<latency>
      mask Display:
      | port_label('input', 1, 'd');
      | port_label('output', 1, 'q');
      | disp(['Z^-', num2str(latency)]);
  we_delay19 : Subsystem  AncestorBlock=casper_library_delays/pipeline  mask(pipeline){latency=3}
      mask help:
      | An explicitly laid-out delay line to avoid mapping to SRL16s
      | for use in pipelining to help achieve timing closure.
      mask init:
      | pipeline_init(gcb,'latency',latency);
      settings: AttributesFormatString=Latency = %<latency>
      mask Display:
      | port_label('input', 1, 'd');
      | port_label('output', 1, 'q');
      | disp(['Z^-', num2str(latency)]);
  we_delay2 : Subsystem  AncestorBlock=casper_library_delays/pipeline  mask(pipeline){latency=3}
      mask help:
      | An explicitly laid-out delay line to avoid mapping to SRL16s
      | for use in pipelining to help achieve timing closure.
      mask init:
      | pipeline_init(gcb,'latency',latency);
      settings: AttributesFormatString=Latency = %<latency>
      mask Display:
      | port_label('input', 1, 'd');
      | port_label('output', 1, 'q');
      | disp(['Z^-', num2str(latency)]);
  we_delay20 : Subsystem  AncestorBlock=casper_library_delays/pipeline  mask(pipeline){latency=15}
      mask help:
      | An explicitly laid-out delay line to avoid mapping to SRL16s
      | for use in pipelining to help achieve timing closure.
      mask init:
      | pipeline_init(gcb,'latency',latency);
      settings: AttributesFormatString=Latency = %<latency>
      mask Display:
      | port_label('input', 1, 'd');
      | port_label('output', 1, 'q');
      | disp(['Z^-', num2str(latency)]);
  we_delay21 : Subsystem  AncestorBlock=casper_library_delays/pipeline  mask(pipeline){latency=15}
      mask help:
      | An explicitly laid-out delay line to avoid mapping to SRL16s
      | for use in pipelining to help achieve timing closure.
      mask init:
      | pipeline_init(gcb,'latency',latency);
      settings: AttributesFormatString=Latency = %<latency>
      mask Display:
      | port_label('input', 1, 'd');
      | port_label('output', 1, 'q');
      | disp(['Z^-', num2str(latency)]);
  we_delay3 : Subsystem  AncestorBlock=casper_library_delays/pipeline  mask(pipeline){latency=3}
      mask help:
      | An explicitly laid-out delay line to avoid mapping to SRL16s
      | for use in pipelining to help achieve timing closure.
      mask init:
      | pipeline_init(gcb,'latency',latency);
      settings: AttributesFormatString=Latency = %<latency>
      mask Display:
      | port_label('input', 1, 'd');
      | port_label('output', 1, 'q');
      | disp(['Z^-', num2str(latency)]);
  we_delay4 : Subsystem  AncestorBlock=casper_library_delays/pipeline  mask(pipeline){latency=3}
      mask help:
      | An explicitly laid-out delay line to avoid mapping to SRL16s
      | for use in pipelining to help achieve timing closure.
      mask init:
      | pipeline_init(gcb,'latency',latency);
      settings: AttributesFormatString=Latency = %<latency>
      mask Display:
      | port_label('input', 1, 'd');
      | port_label('output', 1, 'q');
      | disp(['Z^-', num2str(latency)]);
  we_delay5 : Subsystem  AncestorBlock=casper_library_delays/pipeline  mask(pipeline){latency=3}
      mask help:
      | An explicitly laid-out delay line to avoid mapping to SRL16s
      | for use in pipelining to help achieve timing closure.
      mask init:
      | pipeline_init(gcb,'latency',latency);
      settings: AttributesFormatString=Latency = %<latency>
      mask Display:
      | port_label('input', 1, 'd');
      | port_label('output', 1, 'q');
      | disp(['Z^-', num2str(latency)]);
  we_delay6 : Subsystem  AncestorBlock=casper_library_delays/pipeline  mask(pipeline){latency=3}
      mask help:
      | An explicitly laid-out delay line to avoid mapping to SRL16s
      | for use in pipelining to help achieve timing closure.
      mask init:
      | pipeline_init(gcb,'latency',latency);
      settings: AttributesFormatString=Latency = %<latency>
      mask Display:
      | port_label('input', 1, 'd');
      | port_label('output', 1, 'q');
      | disp(['Z^-', num2str(latency)]);
  we_delay7 : Subsystem  AncestorBlock=casper_library_delays/pipeline  mask(pipeline){latency=3}
      mask help:
      | An explicitly laid-out delay line to avoid mapping to SRL16s
      | for use in pipelining to help achieve timing closure.
      mask init:
      | pipeline_init(gcb,'latency',latency);
      settings: AttributesFormatString=Latency = %<latency>
      mask Display:
      | port_label('input', 1, 'd');
      | port_label('output', 1, 'q');
      | disp(['Z^-', num2str(latency)]);
  we_delay8 : Subsystem  AncestorBlock=casper_library_delays/pipeline  mask(pipeline){latency=3}
      mask help:
      | An explicitly laid-out delay line to avoid mapping to SRL16s
      | for use in pipelining to help achieve timing closure.
      mask init:
      | pipeline_init(gcb,'latency',latency);
      settings: AttributesFormatString=Latency = %<latency>
      mask Display:
      | port_label('input', 1, 'd');
      | port_label('output', 1, 'q');
      | disp(['Z^-', num2str(latency)]);
  we_delay9 : Subsystem  AncestorBlock=casper_library_delays/pipeline  mask(pipeline){latency=3}
      mask help:
      | An explicitly laid-out delay line to avoid mapping to SRL16s
      | for use in pipelining to help achieve timing closure.
      mask init:
      | pipeline_init(gcb,'latency',latency);
      settings: AttributesFormatString=Latency = %<latency>
      mask Display:
      | port_label('input', 1, 'd');
      | port_label('output', 1, 'q');
      | disp(['Z^-', num2str(latency)]);
  " read_addr" : Outport
  wires:
  bank9/1 -> bank7/1  "INT_CALC_fchan"
  bank8/1 -> Terminator6/1  "INT_CALC_accum_ctr"
  bank7/1 -> Terminator7/1  "INT_CALC_xeng"
  Concat1/1 -> Assert6/1, bank8/1, bank9/1  "INT_CALC_addr"
  bank6/1 -> bank2/1  "INT_SLC_fchan"
  bank3/1 -> Terminator4/1  "INT_SLC_accum_ctr"
  bank2/1 -> Terminator5/1  "INT_SLC_xeng"
  we_delay20/1(q) -> Assert7/1, bank6/1, bank3/1  "INT_SLC_addr"
  bank5/1 -> bank1/1  "INT_STR_fchan"
  bank4/1 -> Terminator/1  "INT_STR_accum_ctr"
  bank1/1 -> Terminator3/1  "INT_STR_xeng"
  addr/1 -> Assert2/1  "addr_cntr"
  [addr_slice] -> AddSub2/1
  AddSub2/1 -> Relational/1
  chans_per_x1/1 -> Relational/2
  Relational/1 -> Assertion/1  "BTILC"
  num_x/1 -> Assert3/1
  Assert3/1 -> [num_x]
  chans_per_x_div8/1 -> Assert5/1
  Assert5/1 -> [chans_per_x_div8]
  Assert2/1 -> bank11/1, bank12/1, bank10/1
  bank23/1 -> Concat8/1
  bank25/1 -> Concat8/2
  Concat10/1 -> we_delay20/1(d)
  [fchan_idx] -> bank25/1, bank23/1
  Concat8/1 -> Concat10/3  "spec_reord_SLICE"
  Concat4/1 -> we_delay21/1(d)
  Mult4/1 -> we_delay4/1(d), Mult3/1  "TWO"
  [num_x] -> we_delay1/1(d)
  Mult3/1 -> AddSub3/2
  AddSub3/1 -> Mult5/1  "ONE"
  [addr_calc] -> AddSub2/2
  Assert1/1 -> Concat1/3  "spec_reord_CALC"
  [chans_per_x_div8] -> we_delay2/1(d)
  Mult5/1 -> AddSub4/2
  AddSub4/1 -> Assert1/1
  [bank] -> Concat4/1
  bank10/1 -> [fchan_idx]  "INT_fchan_idx"
  bank12/1 -> [bank]  "INT_bank"
  bank11/1 -> [accum_cnt]  "INT_accum_cnt"
  [fchan_idx] -> we_delay16/1(d), Mult4/1
  [bank] -> Concat10/1
  [accum_cnt] -> Concat10/2
  [one_over_num_x] -> Mult4/2
  one_over_num_x/1 -> Assert4/1
  Assert4/1 -> [one_over_num_x]
  Assert7/1 -> [addr_slice]
  Assert8/1 -> [addr_strght]
  [accum_cnt] -> Concat4/2
  [fchan_idx] -> Concat4/3
  Assert6/1 -> [addr_calc]
  Assert9/1 -> " read_addr"/1
  we_delay16/1(q) -> we_delay5/1(d)
  we_delay1/1(q) -> Mult3/2
  we_delay2/1(q) -> we_delay3/1(d)
  we_delay3/1(q) -> we_delay7/1(d)
  we_delay4/1(q) -> we_delay6/1(d)
  we_delay5/1(q) -> AddSub3/1
  we_delay6/1(q) -> we_delay8/1(d)
  we_delay7/1(q) -> Mult5/2
  we_delay8/1(q) -> AddSub4/1
  [addr_calc] -> Assert9/1
  we_delay21/1(q) -> Assert8/1, bank4/1, bank5/1  "INT_STR_addr"
  out_vec_len/1 -> Terminator2/1
  in_vec_len/1 -> Terminator1/1
  [bank] -> we_delay9/1(d)
  [accum_cnt] -> we_delay10/1(d)
  we_delay9/1(q) -> we_delay12/1(d)
  we_delay10/1(q) -> we_delay11/1(d)
  we_delay11/1(q) -> we_delay14/1(d)
  we_delay12/1(q) -> we_delay13/1(d)
  we_delay13/1(q) -> we_delay17/1(d)
  we_delay14/1(q) -> we_delay15/1(d)
  we_delay15/1(q) -> we_delay19/1(d)
  we_delay17/1(q) -> we_delay18/1(d)
  we_delay18/1(q) -> Concat1/1
  we_delay19/1(q) -> Concat1/2

== system s_c856m4k/hmc_ct/tvg_data_gen ==
  sync : Inport
  dv : Inport  Port=2
  Assert1 : xbsIndex_r4/Assert  assert_type=on  type_source=Explicitly  gui_display_data_type=Boolean  arith_type=Boolean  n_bits=16  bin_pt=14  preci_type=Single  exp_width=8  frac_width=24  assert_rate=on  rate_source=Explicitly  period=1  output_port=on  block_type=assert
  Assert2 : xbsIndex_r4/Assert  assert_type=on  type_source=Explicitly  gui_display_data_type=Boolean  arith_type=Boolean  n_bits=16  bin_pt=14  preci_type=Single  exp_width=8  frac_width=24  assert_rate=on  rate_source=Explicitly  period=1  output_port=on  block_type=assert
  Concat20 : xbsIndex_r4/Concat  num_inputs=4  dbl_ovrd=off  block_type=concat
  Concat21 : xbsIndex_r4/Concat  num_inputs=2  dbl_ovrd=off  block_type=concat
  Delay33 : xbsIndex_r4/Delay  rst=off  infoeditControl=Selection of Reset will increase slice count due to use of real FFs and instead of SRLs  en=off  latency=4  reg_retiming=off  dbl_ovrd=off  block_type=delay
      settings: infoedit=Hardware notes: A delay line is a chain, each link of which is an SRL16 or SRL32 followed by a flip-flop.
  convert_rd_en{,1..3} (4 alike) : xbsIndex_r4/Convert  gui_display_data_type=Fixed-point  arith_type=Unsigned  n_bits=16  bin_pt=0  float_type=Single  exp_bits=8  fraction_bits=24  quantization=Truncate  overflow=Wrap  en=off  latency=0  pipeline=off  dbl_ovrd=off  block_type=convert
      settings: xl_area=[0, 0, 0, 0, 0, 0, 0]
  p0_0 : xbsIndex_r4/Counter  cnt_type=Free Running  cnt_to=Inf  operation=Up  start_count=0  cnt_by_val=4  arith_type=Unsigned  n_bits=input_len_bits + 2  bin_pt=0  load_pin=off  rst=on  en=on  explicit_period=on  period=1  use_behavioral_HDL=off  implementation=Fabric  dbl_ovrd=off  block_type=counter
  p0_1 : xbsIndex_r4/Counter  cnt_type=Free Running  cnt_to=Inf  operation=Up  start_count=1  cnt_by_val=4  arith_type=Unsigned  n_bits=input_len_bits + 2  bin_pt=0  load_pin=off  rst=on  en=on  explicit_period=on  period=1  use_behavioral_HDL=off  implementation=Fabric  dbl_ovrd=off  block_type=counter
  p0_2 : xbsIndex_r4/Counter  cnt_type=Free Running  cnt_to=Inf  operation=Up  start_count=2  cnt_by_val=4  arith_type=Unsigned  n_bits=input_len_bits + 2  bin_pt=0  load_pin=off  rst=on  en=on  explicit_period=on  period=1  use_behavioral_HDL=off  implementation=Fabric  dbl_ovrd=off  block_type=counter
  p0_3 : xbsIndex_r4/Counter  cnt_type=Free Running  cnt_to=Inf  operation=Up  start_count=3  cnt_by_val=4  arith_type=Unsigned  n_bits=input_len_bits + 2  bin_pt=0  load_pin=off  rst=on  en=on  explicit_period=on  period=1  use_behavioral_HDL=off  implementation=Fabric  dbl_ovrd=off  block_type=counter
  d128 : Outport
  wires:
  Delay33/1 -> d128/1
  p0_0/1 -> convert_rd_en/1
  Concat20/1 -> Concat21/2, Concat21/1
  p0_3/1 -> convert_rd_en3/1
  p0_2/1 -> convert_rd_en2/1
  Concat21/1 -> Delay33/1
  convert_rd_en3/1 -> Concat20/4
  convert_rd_en/1 -> Concat20/1
  p0_1/1 -> convert_rd_en1/1
  convert_rd_en2/1 -> Concat20/3
  convert_rd_en1/1 -> Concat20/2
  sync/1 -> Assert2/1
  dv/1 -> Assert1/1
  Assert2/1 -> p0_1/1, p0_2/1, p0_3/1, p0_0/1
  Assert1/1 -> p0_1/2, p0_2/2, p0_3/2, p0_0/2
